simulink model "qube_servo2_quick_start_EE3CL4"  (R2021a)
settings: Solver=ode1  StartTime=0.0  StopTime=5  FixedStep=0.002  RelTol=1e-3  EnableMultiTasking=on
undefined symbols (not defined in the file): HIL, qc_get_step_size
libraries: quarc_library x6, simulink_extras x2, simulink x2
settings Model: EnablePacing=on  PacingRate=0.500000  Creator=amolki  LastModifiedBy=54005
settings SolverCC: AlgebraicLoopSolver=TrustRegion
settings DebuggingCC: SFMachineParentedDataDiag=warning
settings SFSimCC: CustomCodeUndefinedFunction=UseInterfaceOnly

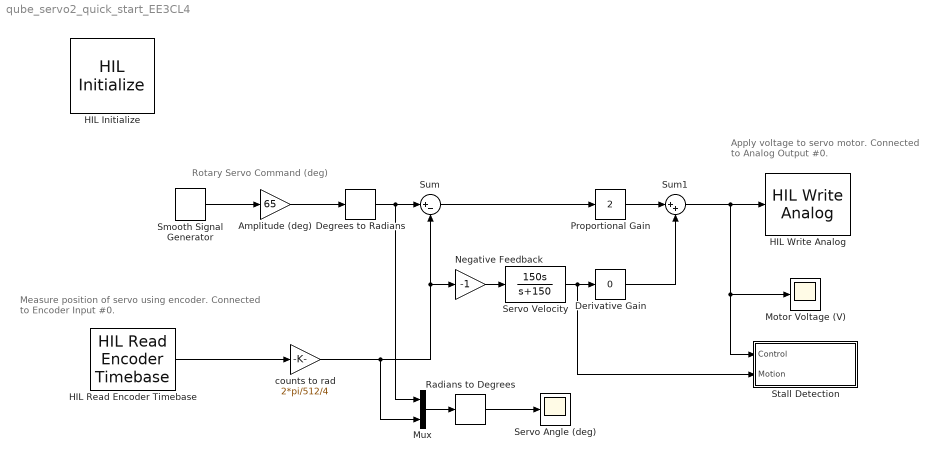
== system qube_servo2_quick_start_EE3CL4 ==
  note: Rotary Servo Command (deg)
  note: Measure position of servo using encoder.
      | Connected to Encoder Input #0.
  note: Apply voltage to servo motor.
      | Connected to Analog Output #0.
  Amplitude (deg) : Gain  Gain=65
  Degrees to Radians : simulink_extras/Transformations/Degrees to Radians
  Derivative Gain : simulink/Math Operations/Slider Gain  gain=0  low=0  high=0.5
  HIL Initialize : quarc_library/Data Acquisition/Generic/Configuration/HIL Initialize  Priority=-99  object_name=HIL-1  board_type=qube_servo2_usb  board_number=0@tcpip://localhost:18920  board_options=d0=digital;d1=digital;led=auto;update_rate=normal;decimation=1  exclusive=off  active=on  hardware_clocks=[0]  clock_modes=[]  initial_clock_frequencies=[]  set_clock_params_at_start=off  set_clock_params_at_switch_in=off  set_clock_frequencies_at_start=off  set_clock_frequencies_at_switch_in=off  analog_input_channels=[0]  analog_input_configurations=[]  analog_input_maximums=3  analog_input_minimums=-3  set_analog_input_params_at_start=off  set_analog_input_params_at_switch_in=off  analog_output_channels=[0]  analog_output_maximums=15  analog_output_minimums=-15  initial_analog_outputs=[0]  final_analog_outputs=[0]  watchdog_analog_outputs=0  set_analog_output_params_at_start=off  set_analog_output_params_at_switch_in=off  set_analog_outputs_at_start=on  set_analog_outputs_at_switch_in=off  set_analog_outputs_at_terminate=on  set_analog_outputs_at_switch_out=off  set_analog_outputs_on_watchdog=on  digital_input_channels=[]  digital_output_channels=[0]  digital_output_configuration=[]  initial_digital_outputs=[1]  final_digital_outputs=[0]  watchdog_digital_outputs=[0]  set_digital_output_params_at_start=off  set_digital_output_params_at_switch_in=off  set_digital_outputs_at_start=on  set_digital_outputs_at_switch_in=off  set_digital_outputs_at_terminate=on  set_digital_outputs_at_switch_out=off  set_digital_outputs_on_watchdog=on  encoder_channels=[0:1]  quadrature=[4]  encoder_filter_frequency=[]  initial_encoder_counts=[0]  set_encoder_params_at_start=off  set_encoder_params_at_switch_in=off  set_encoder_counts_at_start=on  set_encoder_counts_at_switch_in=off  pwm_channels=[]  pwm_modes=[]  pwm_frequency=[]  pwm_configuration=[]  pwm_alignment=[]  pwm_polarity=[]  pwm_leading_deadband=[]  pwm_trailing_deadband=[]  initial_pwm_outputs=[]  final_pwm_outputs=[]  watchdog_pwm_outputs=[]  set_pwm_params_at_start=off  set_pwm_params_at_switch_in=off  set_pwm_outputs_at_start=off  set_pwm_outputs_at_switch_in=off  set_pwm_outputs_at_terminate=off  set_pwm_outputs_at_switch_out=off  set_pwm_outputs_on_watchdog=off  other_output_channels=[11000:11002]  initial_other_outputs=[0 1 0]  final_other_outputs=[1 0 0]  watchdog_other_outputs=[0 0 1]  set_other_outputs_at_start=on  set_other_outputs_at_switch_in=off  set_other_outputs_at_terminate=on  set_other_outputs_at_switch_out=off  set_other_outputs_on_watchdog=on
  HIL Read Encoder Timebase : quarc_library/Data Acquisition/Generic/Timebases/HIL Read Encoder Timebase  object_name=HIL-1  clock=0  channels=0  active=on  vector_output=off  data_type_mode=Inherit via back propagation  data_type=double  overflow_mode=Synchronize (for simulated cards only)  samples_in_buffer=1+0*max(ceil(1/qc_get_step_size), 1)
  HIL Write Analog : quarc_library/Data Acquisition/Generic/Immediate I//O/HIL Write Analog  object_name=HIL-1  channels=0  sample_time=-1  active=on  vector_input=off
  Motor Voltage (V) : Scope
  Mux : Mux  Inputs=2
  Negative Feedback : Gain  Gain=-1
  Proportional Gain : simulink/Math Operations/Slider Gain  gain=2  low=0  high=10
  Radians to Degrees : simulink_extras/Transformations/Radians to Degrees
  Servo Angle (deg) : Scope
  Servo Velocity : TransferFcn  Numerator=[150 0]  Denominator=[1 150]
  Smooth Signal Generator : quarc_library/Sources/Signals/Smooth Signal Generator  signal_type=Square  source=Internal (dialog parameters)  amplitude=0.6923  frequency=0.4  initial_phase=0  sample_time=qc_get_step_size  output_cos=off
      settings: SourceProductName=QUARC Targets
  Stall Detection : Subsystem
  Sum : Sum  Inputs=|+-
  Sum1 : Sum  Inputs=|++
  counts to rad : Gain  Gain=2*pi/512/4
  wires:
  Amplitude (deg)/1 -> Degrees to Radians/1
  Smooth Signal Generator/1 -> Amplitude (deg)/1
  Servo Velocity/1 -> Stall Detection/2(Motion), Derivative Gain/1
  counts to rad/1 -> Sum/2, Negative Feedback/1, Mux/2
  Derivative Gain/1 -> Sum1/2
  Sum1/1 -> HIL Write Analog/1, Stall Detection/1(Control), Motor Voltage (V)/1
  Radians to Degrees/1 -> Servo Angle (deg)/1
  Mux/1 -> Radians to Degrees/1
  Proportional Gain/1 -> Sum1/1
  Degrees to Radians/1 -> Sum/1, Mux/1
  HIL Read Encoder Timebase/1 -> counts to rad/1
  Negative Feedback/1 -> Servo Velocity/1
  Sum/1 -> Proportional Gain/1

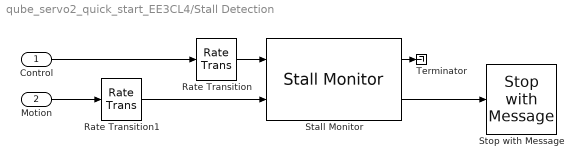
== system qube_servo2_quick_start_EE3CL4/Stall Detection ==
  Control : Inport
  Motion : Inport  Port=2
  Rate Transition : RateTransition
  Rate Transition1 : RateTransition
  Stall Monitor : quarc_library/Discrete/Stall Monitor  control_threshold=5  motion_threshold=0.3  duration_s=20
      settings: SourceProductName=QUARC Targets
  Stop with Message : quarc_library/Sinks/Error Handling/Stop with Message  message_type=Fixed error message  message_icon=Error  message=Stall Detected! Please ensure that the DC motor is free to move and is functioning properly
  Terminator : Terminator
  wires:
  Control/1 -> Rate Transition/1
  Motion/1 -> Rate Transition1/1
  Stall Monitor/2 -> Stop with Message/1
  Stall Monitor/1 -> Terminator/1
  Rate Transition/1 -> Stall Monitor/1
  Rate Transition1/1 -> Stall Monitor/2
